simulink model "NonLinearPatient"  (R2022a)
settings: Solver=VariableStepAuto  StartTime=0.0  StopTime=10.0  RelTol=1e-3
values from neighbouring files (symbols this model uses):
  contDiscMat = BuildCondendsedMPCmatrices(discreteMat,r,q,F,f,PH)    [nonLinearPatient_main.m]
  PH = 200    [MAIN_MIMO.m]    (also in backupMain.m; nonLinearPatient_main.m; test.m)
  R_KF = 0.001*eye(2)    [MAIN_MIMO.m]    (also in backupMain.m; nonLinearPatient_main.m; test.m)
  u_eq = [propofol_eq; remifentanil_eq]    [MAIN_MIMO.m]    (also in backupMain.m; nonLinearPatient_main.m; test.m)
  wantNoisyBIS = 1    [MAIN_MIMO.m]    (also in backupMain.m; nonLinearPatient_main.m; test.m)
  x_eq = operatingPoint.getstatestruct.signals.values    [MAIN_MIMO.m]    (also in backupMain.m; nonLinearPatient_main.m; test.m)
undefined symbols (not defined in the file or in its folder): Discrete, info, myMPC_dist, op, patient, propofol, RASS, remifentanil, Time
libraries: cstblocks x2, ctrlSharedLib x1
settings Model: Creator=user  LastModifiedBy=user

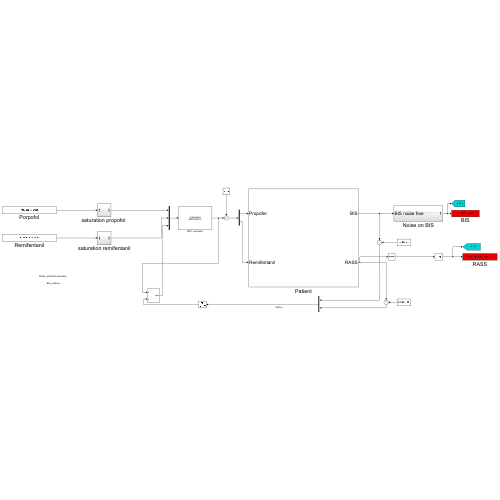
[thumbnail: Simulink's stored preview of the top-level diagram]
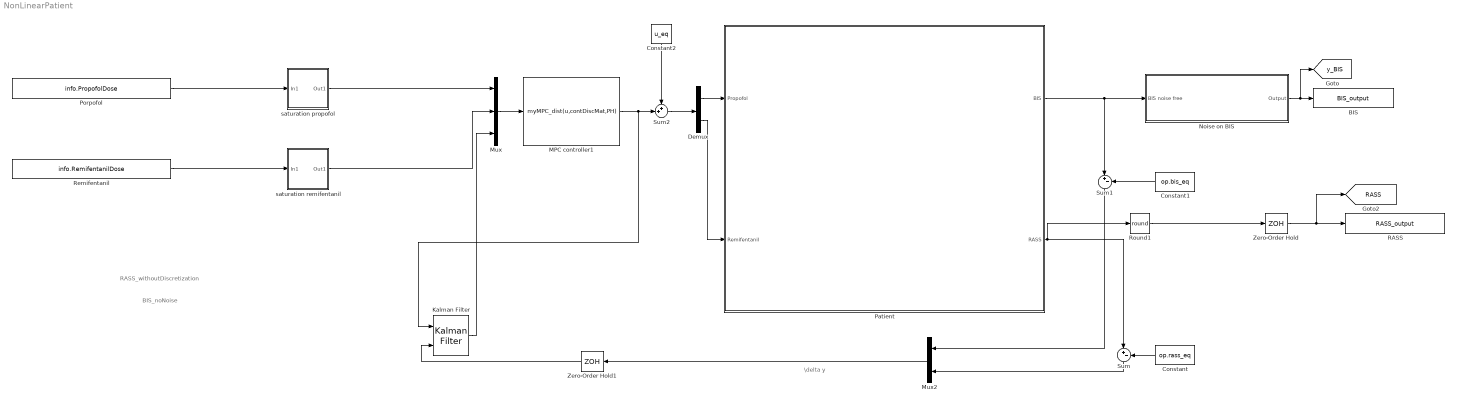
== system NonLinearPatient ==
  note: \delta y
  note: RASS_withoutDiscretization
  note: BIS_noNoise
  BIS : ToWorkspace  VariableName=BIS_output  SaveFormat=Structure With Time  SampleTime=info.Ts
      settings: Save2DSignal=2-D array (concatenate along first dimension)
  Constant : Constant  Value=op.rass_eq
  Constant1 : Constant  Value=op.bis_eq
  Constant2 : Constant  Value=u_eq
  Demux : Demux  Outputs=2
  Kalman Filter : ctrlSharedLib/Kalman Filter  TimeDomain=Discrete-Time  UseCurrentEstimator=on  ModelSource=LTI State-Space Variable  ModelSourceVariable=discreteModel  A=0.95  B=1  C=1  D=0  NumberOfStates=1  NumberOfInputs=1  NumberOfOutputs=1  InitialEstimateSource=Dialog  X0=x_eq  P0=10  UseK=off  UseGH=off  NumberOfProcessNoiseInputs=1  G=1  TimeInvariantG=on  H=0  TimeInvariantH=on  Q=Q_KF  TimeInvariantQ=on  R=R_KF  TimeInvariantR=on  N=0  TimeInvariantN=on  AddInputPort=on  AddEnablePort=off  OutputEstimatedY=off  OutputP=off  Ts=-1
  MPC controller1 : MATLABFcn  MATLABFcn=myMPC_dist(u,contDiscMat,PH)  OutputDimensions=2
  Mux : Mux  Inputs=3
  Mux2 : Mux  Inputs=2
  Noise on BIS : Subsystem
  Patient : Subsystem
  Porpofol : Constant  Value=info.PropofolDose  SampleTime=info.Ts
  RASS : ToWorkspace  VariableName=RASS_output  SaveFormat=Structure With Time  SampleTime=info.Ts
      settings: Save2DSignal=2-D array (concatenate along first dimension)
  Remifentanil : Constant  Value=info.RemifentanilDose  SampleTime=info.Ts
  Round1 : Rounding  Operator=round
  Sum : Sum  Inputs=|+-
  Sum1 : Sum  Inputs=|+-
  Sum2 : Sum  Inputs=++|
  Zero-Order Hold : ZeroOrderHold  SampleTime=info.Ts
  Zero-Order Hold1 : ZeroOrderHold
  "saturation propofol " : Subsystem
  saturation remifentanil : Subsystem
  tag scope: RASS=global, y_BIS=global
  wires:
  Demux/1 -> Patient/1(Propofol)
  Constant1/1 -> Sum1/2
  Mux2/1 -> Zero-Order Hold1/1
  Sum/1 -> Mux2/2
  saturation remifentanil/1(Out1) -> Mux/2
  Sum1/1 -> Mux2/1
  Demux/2 -> Patient/2(Remifentanil)
  Constant/1 -> Sum/2
  Kalman Filter/1 -> Mux/3
  Mux/1 -> MPC controller1/1
  Porpofol/1 -> "saturation propofol "/1(In1)
  Remifentanil/1 -> saturation remifentanil/1(In1)
  Round1/1 -> Zero-Order Hold/1
  "saturation propofol "/1(Out1) -> Mux/1
  Noise on BIS/1(Output) -> BIS/1, [y_BIS]
  Patient/2(RASS) -> Sum/1, Round1/1
  Patient/1(BIS) -> Noise on BIS/1(BIS noise free), Sum1/1
  Zero-Order Hold/1 -> RASS/1, [RASS]
  MPC controller1/1 -> Kalman Filter/1, Sum2/2
  Constant2/1 -> Sum2/1
  Sum2/1 -> Demux/1
  Zero-Order Hold1/1 -> Kalman Filter/2

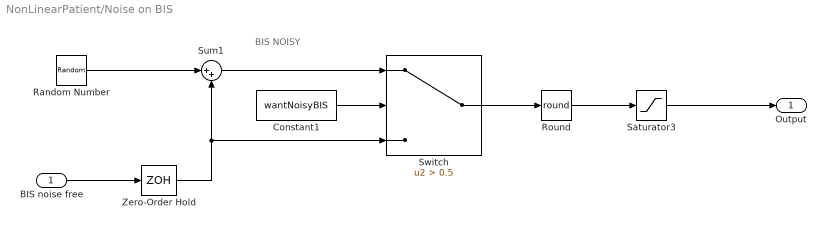
== system NonLinearPatient/Noise on BIS ==
  note: BIS NOISY
  BIS noise free : Inport
  Constant1 : Constant  Value=wantNoisyBIS
  Random Number : RandomNumber  Variance=6.27  SampleTime=info.Ts
  Round : Rounding  Operator=round
  Saturator3 : Saturate  UpperLimit=100  LowerLimit=0
  Sum1 : Sum  Inputs=|++
  Switch : Switch  Criteria=u2 > Threshold  Threshold=0.5  SaturateOnIntegerOverflow=off  InputSameDT=off
  Zero-Order Hold : ZeroOrderHold  SampleTime=info.Ts
  Output : Outport
  wires:
  Round/1 -> Saturator3/1
  Random Number/1 -> Sum1/1
  Constant1/1 -> Switch/2
  Saturator3/1 -> Output/1
  Switch/1 -> Round/1
  BIS noise free/1 -> Zero-Order Hold/1
  Sum1/1 -> Switch/1
  Zero-Order Hold/1 -> Sum1/2, Switch/3

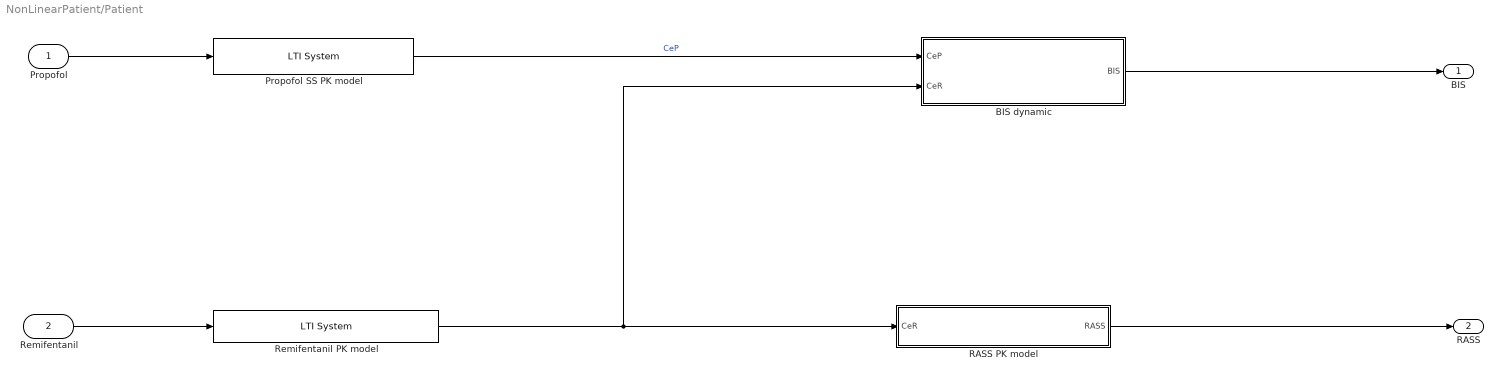
== system NonLinearPatient/Patient ==
  Propofol : Inport
  Remifentanil : Inport  Port=2
  BIS dynamic : Subsystem
  Propofol SS PK model : cstblocks/LTI System  sys=propofol.propSS  IC=0
  RASS PK model : Subsystem
  Remifentanil PK model : cstblocks/LTI System  sys=remifentanil.remiSS  IC=0
  BIS : Outport
  RASS : Outport  Port=2
  wires:
  Propofol SS PK model/1 -> BIS dynamic/1(CeP)  "CeP"
  BIS dynamic/1(BIS) -> BIS/1
  Propofol/1 -> Propofol SS PK model/1
  Remifentanil/1 -> Remifentanil PK model/1
  Remifentanil PK model/1 -> RASS PK model/1(CeR), BIS dynamic/2(CeR)
  RASS PK model/1(RASS) -> RASS/1

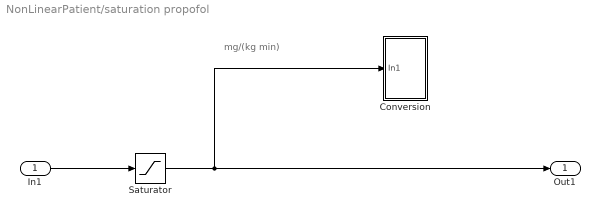
== system NonLinearPatient/saturation propofol  ==
  note: mg/(kg min)
  In1 : Inport
  Conversion : Subsystem
  Saturator : Saturate  UpperLimit=5  LowerLimit=0
  Out1 : Outport
  wires:
  In1/1 -> Saturator/1
  Saturator/1 -> Out1/1, Conversion/1(In1)

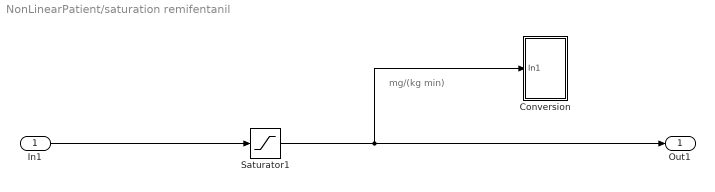
== system NonLinearPatient/saturation remifentanil ==
  note: mg/(kg min)
  In1 : Inport
  "Conversion " : Subsystem
  Saturator1 : Saturate  UpperLimit=2.5  LowerLimit=0
  Out1 : Outport
  wires:
  In1/1 -> Saturator1/1
  Saturator1/1 -> Out1/1, "Conversion "/1(In1)

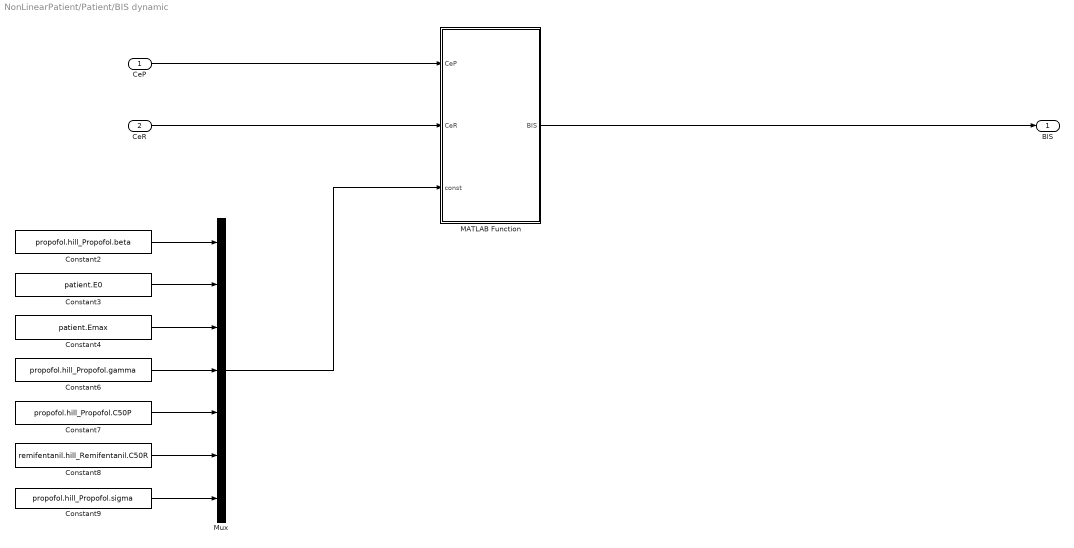
== system NonLinearPatient/Patient/BIS dynamic ==
  CeP : Inport
  CeR : Inport  Port=2
  Constant2 : Constant  Value=propofol.hill_Propofol.beta
  Constant3 : Constant  Value=patient.E0
  Constant4 : Constant  Value=patient.Emax
  Constant6 : Constant  Value=propofol.hill_Propofol.gamma
  Constant7 : Constant  Value=propofol.hill_Propofol.C50P
  Constant8 : Constant  Value=remifentanil.hill_Remifentanil.C50R
  Constant9 : Constant  Value=propofol.hill_Propofol.sigma
  MATLAB Function : MATLAB Function  TreatAsAtomicUnit=on
  Mux : Mux  Inputs=7
  BIS : Outport
  wires:
  Constant9/1 -> Mux/7
  Constant8/1 -> Mux/6
  Constant4/1 -> Mux/3
  Mux/1 -> MATLAB Function/3(const)
  Constant7/1 -> Mux/5
  Constant3/1 -> Mux/2
  Constant6/1 -> Mux/4
  Constant2/1 -> Mux/1
  MATLAB Function/1(BIS) -> BIS/1
  CeP/1 -> MATLAB Function/1(CeP)
  CeR/1 -> MATLAB Function/2(CeR)

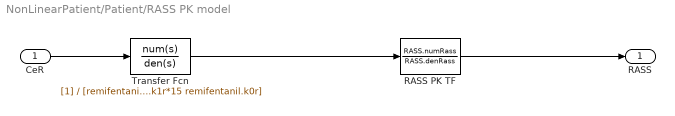
== system NonLinearPatient/Patient/RASS PK model ==
  CeR : Inport
  RASS PK TF : TransferFcn  Numerator=RASS.numRass  Denominator=RASS.denRass
  Transfer Fcn : TransferFcn  Denominator=[remifentanil.k1r*15 remifentanil.k0r]
  RASS : Outport
  wires:
  CeR/1 -> Transfer Fcn/1
  Transfer Fcn/1 -> RASS PK TF/1
  RASS PK TF/1 -> RASS/1

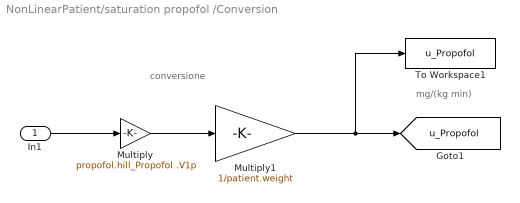
== system NonLinearPatient/saturation propofol /Conversion ==
  note: mg/(kg min)
  note: conversione
  In1 : Inport
  Multiply : Gain  Gain=propofol.hill_Propofol .V1p
  Multiply1 : Gain  Gain=1/patient.weight
  To Workspace1 : ToWorkspace  VariableName=u_Propofol  SaveFormat=Structure With Time  SampleTime=-1
      settings: Save2DSignal=2-D array (concatenate along first dimension)
  tag scope: u_Propofol=global
  wires:
  In1/1 -> Multiply/1
  Multiply/1 -> Multiply1/1
  Multiply1/1 -> To Workspace1/1, [u_Propofol]

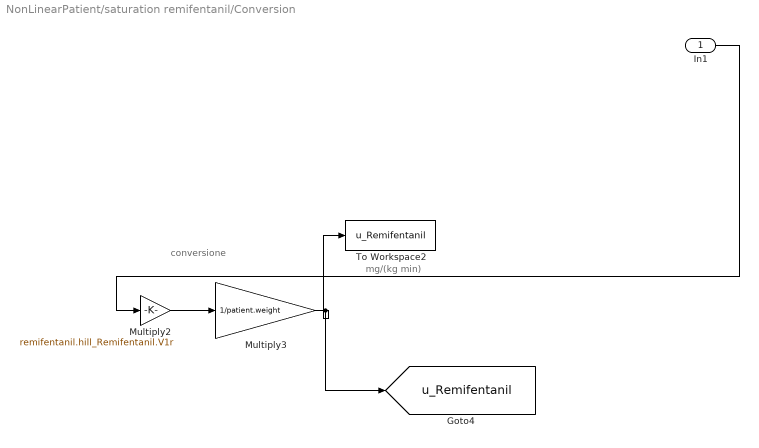
== system NonLinearPatient/saturation remifentanil/Conversion  ==
  note: mg/(kg min)
  note: conversione
  In1 : Inport
  Multiply2 : Gain  Gain=remifentanil.hill_Remifentanil.V1r
  Multiply3 : Gain  Gain=1/patient.weight
  To Workspace2 : ToWorkspace  VariableName=u_Remifentanil  SaveFormat=Structure With Time  SampleTime=-1
      settings: Save2DSignal=2-D array (concatenate along first dimension)
  tag scope: u_Remifentanil=global
  wires:
  Multiply2/1 -> Multiply3/1
  In1/1 -> Multiply2/1
  Multiply3/1 -> To Workspace2/1, [u_Remifentanil]

== matlab function NonLinearPatient/Patient/BIS dynamic/MATLAB Function ==
  data: CeP input; BIS output; CeR input; const input
function BIS = fcn(CeP,CeR, const)

if CeP >=0 && CeR >=0
    %% Constant declaration
    beta = const(1);
    E0 = const(2); %starting effect
%     E0 = const(2)-100; %starting effect
    Emax = const(3); %maximum effect achievable
    gamma = const(4); %sigmoidicity
    C50P = const(5); % half effect concentration
    C50R = const(6); % half effect concentration
    sigma = const(7);% sinergy between prop & rem
    
    %% 2D Calculations
    Uprop=CeP./C50P; Uremi=CeR./C50R;
    BIS=E0 - Emax*((Uprop)+(Uremi)+sigma*(Uprop)*(Uremi))^(gamma)/...
        (1+(Uprop+Uremi+sigma*Uprop*Uremi)^(gamma));

else
    BIS = 100;
end
